simulink model "MPC_PMM_ph_gaslift"  (R2023a)
settings: Solver=ode15s  StartTime=0.0  StopTime=par.simulation_time  FixedStep=par.sample_time  RelTol=1e-3
values from neighbouring files (symbols this model uses):
  A = blkdiag(plant_discrete.A, plant_output_disturbance.A)    [main_MPC_PMM_ph_gaslift.m]
  Bu = [plant_discrete.B; 0]    [main_MPC_PMM_ph_gaslift.m]
  Cm = [plant_discrete.C, plant_output_disturbance.C]    [main_MPC_PMM_ph_gaslift.m]
  par = function_parameters_MPC_PMM_ph_gaslift    [main_MPC_PMM_ph_gaslift.m]
  u0 = operating_report.Inputs.u    [main_MPC_PMM_ph_gaslift.m]
  x0 = [operating_report.States(1).x; operating_report.States(2).x]    [main_MPC_PMM_ph_gaslift.m]
  y0 = operating_report.Outputs.y    [main_MPC_PMM_ph_gaslift.m]
undefined symbols (not defined in the file or in its folder): L, M
libraries: mpclib x1
settings Model: ExtModeTrigMode=oneshot  Creator=The MathWorks, Inc.  LastModifiedBy=aslik
settings SolverCC: ZeroCrossControl=DisableAll  ZeroCrossAlgorithm=Adaptive  AlgebraicLoopSolver=TrustRegion
settings DataIOCC: InspectSignalLogs=on  ReturnWorkspaceOutputs=off  DatasetSignalFormat=timetable
settings OptimizationCC: BooleanDataType=off  DefaultParameterBehavior=Inlined  EnhancedBackFolding=on  PassReuseOutputArgsAs=Individual arguments  ExpressionDepthLimit=2147483647  ZeroExternalMemoryAtStartup=off  ZeroInternalMemoryAtStartup=off  InitFltsAndDblsToZero=on  OptimizeBlockOrder=speed  DifferentSizesBufferReuse=on  OptimizationCustomize=off  EfficientTunableParamExpr=on
settings DebuggingCC: UnderspecifiedInitializationDetection=Classic  MergeDetectMultiDrivingBlocksExec=none  CheckExecutionContextPreStartOutputMsg=on  SignalResolutionControl=TryResolveAllWithWarning  IgnoredZcDiagnostic=none  MultiTaskDSMMsg=warning  MultiTaskCondExecSysMsg=none  IntegerOverflowMsg=none  ParameterTunabilityLossMsg=error  FcnCallInpInsideContextMsg=warning  UnconnectedInputMsg=warning  UnconnectedOutputMsg=warning  UnconnectedLineMsg=warning  StateNameClashWarn=warning  SFUnexpectedBacktrackingDiag=warning  SFNoUnconditionalDefaultTransitionDiag=warning  SFExecutionAtInitializationDiag=none  IntegerSaturationMsg=none  ArithmeticOperatorsInVariantConditions=warning
settings HardwareCC: TargetBitPerPointer=64  TargetBitPerSizeT=64  TargetBitPerPtrDiffT=64  TargetLongLongMode=on  TargetIntDivRoundTo=Zero  TargetEndianess=LittleEndian  TargetWordSize=64  TargetHWDeviceType=MATLAB Host  ProdEqTarget=off
settings ModelReferenceCC: EnableRefExpFcnMdlSchedulingChecks=on  PropagateSignalLabelsOutOfModel=off
settings SFSimCC: SimUseLocalCustomCode=off  MATLABDynamicMemAlloc=off  CustomCodeUndefinedFunction=UseInterfaceOnly
settings RTWCC: Description=Embedded Coder  SystemTargetFile=ert.tlc  TemplateMakefile=ert_default_tmf  RTWUseLocalCustomCode=off  DLArmComputeVersion=19.05
settings CodeAppCC: ForceParamTrailComments=on  IgnoreCustomStorageClasses=off  OperatorAnnotations=on  SimulinkDataObjDesc=on  SFDataObjDesc=on  InsertBlockDesc=on
settings ERTTargetCC: GenerateSampleERTMain=on  InlinedParameterPlacement=NonHierarchical  ERTCustomFileTemplate=example_file_process.tlc
settings ConfigComp: CovMetricSettings=dw  CovSaveCumulativeToWorkspaceVar=on  CovSaveSingleToWorkspaceVar=on  CovExternalEMLEnable=off  CovSFcnEnable=off

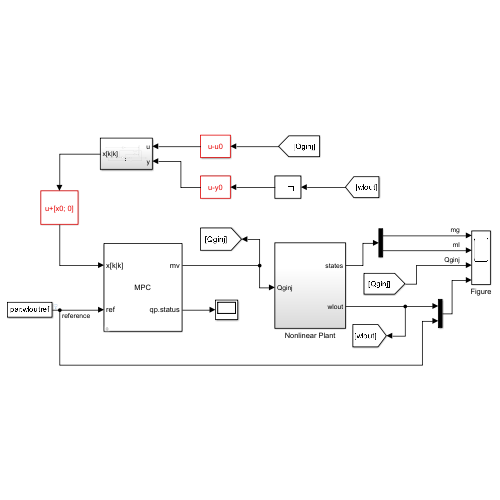
[thumbnail: Simulink's stored preview of the top-level diagram]
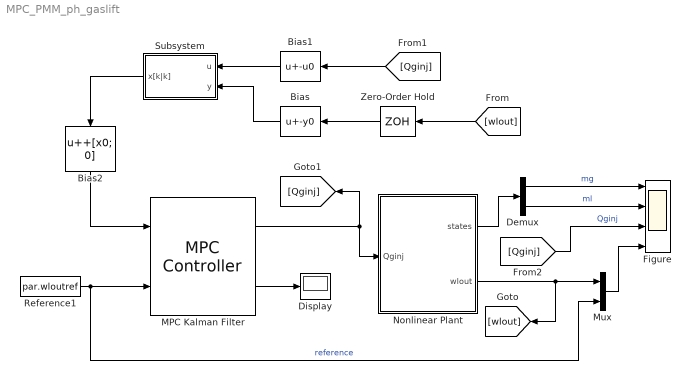
== system MPC_PMM_ph_gaslift ==
  Bias : Bias  Bias=-y0  SaturateOnIntegerOverflow=off
  Bias1 : Bias  Bias=-u0  SaturateOnIntegerOverflow=off
  Bias2 : Bias  Bias=+[x0; 0]  SaturateOnIntegerOverflow=off
  Demux : Demux  Outputs=2
  Display : Display
  Figure : Scope  NumInputPorts=4
  MPC Kalman Filter : mpclib/MPC Controller  mpcobj=mpcobj  x0=[]  is_multiple=0  enable_value=0  return_u0=off  updateMPCinCallerWorkspace=on  md_inport=off  mv_inport=off  uref_inport=off  return_cost=off  return_mvseq=off  return_qpstatus=on  return_xseq=off  return_state=off  return_ovseq=off  state_inport=on  umin_inport=off  umax_inport=off  ymin_inport=off  ymax_inport=off  cc_inport=off  ywt_inport=off  uwt_inport=off  duwt_inport=off  rhoeps_inport=off  pm_inport=off  MaximumP=10  HorizonChoice=FixedHorizon  n_ts=0.01  n_p=10  n_mv=1  n_md=0  n_ud=0  n_mo=1  n_uo=0  BlockDataType=double  SampleTimeInherited=off  switch_inport=off
  Mux : Mux  Inputs=2
  Nonlinear Plant : Subsystem
  Reference1 : Constant  Value=par.wloutref  SampleTime=0
  Subsystem : Subsystem
  Zero-Order Hold : ZeroOrderHold  SampleTime=par.sample_time
  wires:
  Bias/1 -> Subsystem/2(y)
  Nonlinear Plant/2(wlout) -> [wlout], Mux/1
  Reference1/1 -> MPC Kalman Filter/2, Mux/2  "reference"
  Bias2/1 -> MPC Kalman Filter/1
  Bias1/1 -> Subsystem/1(u)
  MPC Kalman Filter/1 -> Nonlinear Plant/1(Qginj), [Qginj]
  Zero-Order Hold/1 -> Bias/1
  Subsystem/1(x[k|k]) -> Bias2/1
  [Qginj] -> Figure/3  "Qginj"
  [Qginj] -> Bias1/1
  Nonlinear Plant/1(states) -> Demux/1
  Demux/2 -> Figure/2  "ml"
  Demux/1 -> Figure/1  "mg"
  [wlout] -> Zero-Order Hold/1
  Mux/1 -> Figure/4
  MPC Kalman Filter/2 -> Display/1

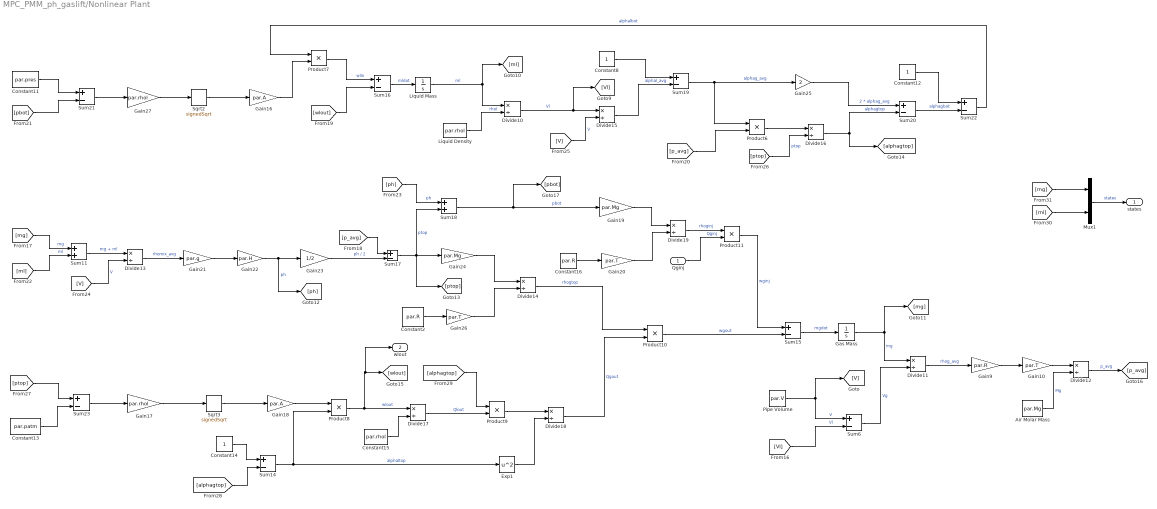
== system MPC_PMM_ph_gaslift/Nonlinear Plant ==
  Qginj : Inport
  Air Molar Mass : Constant  Value=par.Mg  OutDataTypeStr=double
  Constant11 : Constant  Value=par.pres  OutDataTypeStr=double
  Constant12 : Constant  OutDataTypeStr=double
  Constant13 : Constant  Value=par.patm  OutDataTypeStr=double
  Constant14 : Constant  OutDataTypeStr=double
  Constant15 : Constant  Value=par.rhol  OutDataTypeStr=double
  Constant16 : Constant  Value=par.R  OutDataTypeStr=double
  Constant2 : Constant  Value=par.R  OutDataTypeStr=double
  Constant8 : Constant  OutDataTypeStr=double
  Divide{10..19} (10 alike) : Product  Inputs=*/
  Exp1 : Math  Operator=square
  Gain10 : Gain  Gain=par.T
  Gain16 : Gain  Gain=par.A
  Gain17 : Gain  Gain=par.rhol
  Gain18 : Gain  Gain=par.A
  Gain19 : Gain  Gain=par.Mg
  Gain20 : Gain  Gain=par.T
  Gain21 : Gain  Gain=par.g
  Gain22 : Gain  Gain=par.H
  Gain23 : Gain  Gain=1/2
  Gain24 : Gain  Gain=par.Mg
  Gain25 : Gain  Gain=2
  Gain26 : Gain  Gain=par.T
  Gain27 : Gain  Gain=par.rhol
  Gain9 : Gain  Gain=par.R
  "Gas Mass " : Integrator  InitialCondition=x0(1)  LowerSaturationLimit=0  ContinuousStateAttributes='mg'
  Liquid Density : Constant  Value=par.rhol  OutDataTypeStr=double
  Liquid Mass : Integrator  InitialCondition=x0(2)  LowerSaturationLimit=0  ContinuousStateAttributes='ml'
  Mux1 : Mux  Inputs=2
  Pipe Volume : Constant  Value=par.V  OutDataTypeStr=double
  Product{6..11} (6 alike) : Product
  Sqrt2 : Sqrt  Operator=signedSqrt
  Sqrt3 : Sqrt  Operator=signedSqrt
  Sum11 : Sum
  Sum{6,14..17,19..23} (10 alike) : Sum  Inputs=+-
  Sum18 : Sum
  states : Outport
  wlout : Outport  Port=2
  wires:
  Liquid Mass/1 -> [ml], Divide10/1  "ml"
  Constant13/1 -> Sum23/2
  Sum6/1 -> Divide11/2  "Vg"
  Sum11/1 -> Divide13/1  "mg + ml"
  Gain18/1 -> Product8/1
  Product7/1 -> Sum16/1  "wlin"
  Product10/1 -> Sum15/2  "wgout"
  "Gas Mass "/1 -> [mg], Divide11/1  "mg"
  Gain22/1 -> [ph], Gain23/1  "ph"
  [mg] -> Sum11/1  "mg"
  [ml] -> Sum11/2  "ml"
  Sqrt2/1 -> Gain16/1
  [wlout] -> Sum16/2
  [V] -> Divide13/2  "V"
  Air Molar Mass/1 -> Divide12/2  "Mg"
  Sum18/1 -> [pbot], Gain19/1  "pbot"
  Divide19/1 -> Product11/1  "rhoginj"
  Product9/1 -> Divide18/1
  Sum20/1 -> Sum22/2  "alphagbot"
  [pbot] -> Sum21/2
  Constant2/1 -> Gain26/1
  Liquid Density/1 -> Divide10/2  "rhol"
  Sqrt3/1 -> Gain18/1
  Sum19/1 -> Product6/1, Gain25/1  "alphag_avg"
  [ptop] -> Divide16/2  "ptop"
  Constant12/1 -> Sum22/1
  Qginj/1 -> Product11/2  "Qginj"
  [alphagtop] -> Product9/1
  Sum15/1 -> "Gas Mass "/1  "mgdot"
  Gain24/1 -> Divide14/1
  Gain23/1 -> Sum17/2  "ph / 2"
  [p_avg] -> Sum17/1
  [Vl] -> Sum6/2  "Vl"
  Sum21/1 -> Gain27/1
  Divide18/1 -> Product10/2  "Qgout"
  Gain9/1 -> Gain10/1
  Divide13/1 -> Gain21/1  "rhomix_avg"
  Gain27/1 -> Sqrt2/1
  Gain26/1 -> Divide14/2
  Exp1/1 -> Divide18/2
  Product11/1 -> Sum15/1  "wginj"
  Gain25/1 -> Sum20/1  "2 * alphag_avg"
  Pipe Volume/1 -> [V], Sum6/1  "V"
  [p_avg] -> Product6/2
  Constant11/1 -> Sum21/1
  Gain10/1 -> Divide12/1
  Gain20/1 -> Divide19/2
  Sum17/1 -> Gain24/1, Sum18/2, [ptop]  "ptop"
  Sum14/1 -> Product8/2, Exp1/1  "alphaltop"
  Divide15/1 -> Sum19/2  "alphal_avg"
  Gain19/1 -> Divide19/1
  Product6/1 -> Divide16/1
  Divide12/1 -> [p_avg]  "p_avg"
  Gain16/1 -> Product7/2
  Product8/1 -> wlout/1, [wlout], Divide17/1  "wlout"
  Constant14/1 -> Sum14/1
  [ml] -> Mux1/2
  Sum23/1 -> Gain17/1
  Constant15/1 -> Divide17/2
  [mg] -> Mux1/1
  Divide11/1 -> Gain9/1  "rhog_avg"
  Mux1/1 -> states/1  "states"
  Divide14/1 -> Product10/1  "rhogtop"
  Sum16/1 -> Liquid Mass/1  "mldot"
  [V] -> Divide15/2  "V"
  [alphagtop] -> Sum14/2
  Gain17/1 -> Sqrt3/1
  Gain21/1 -> Gain22/1
  Constant8/1 -> Sum19/1
  Constant16/1 -> Gain20/1
  Divide17/1 -> Product9/2  "Qlout"
  [ph] -> Sum18/1  "ph"
  Divide16/1 -> [alphagtop], Sum20/2  "alphagtop"
  Divide10/1 -> Divide15/1, [Vl]  "Vl"
  Sum22/1 -> Product7/1  "alphalbot"
  [ptop] -> Sum23/1

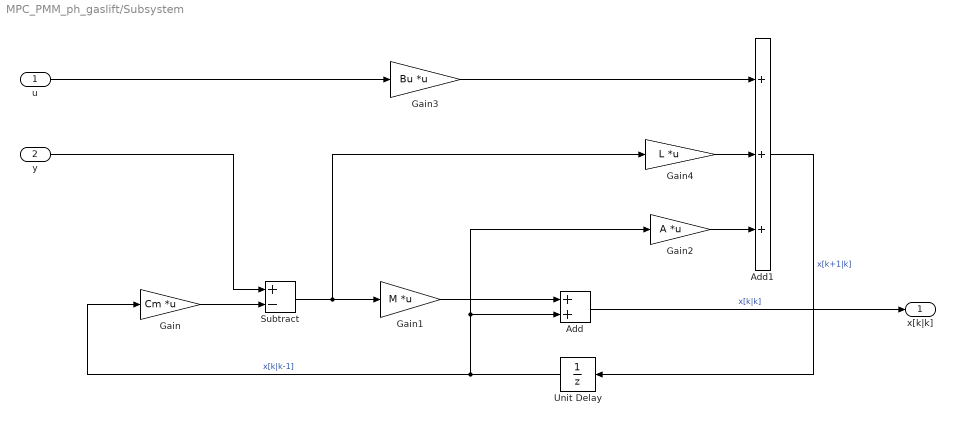
== system MPC_PMM_ph_gaslift/Subsystem ==
  u : Inport
  y : Inport  Port=2
  Add : Sum
  Add1 : Sum  Inputs=+++
  Gain : Gain  Gain=Cm  Multiplication=Matrix(K*u)
  Gain1 : Gain  Gain=M  Multiplication=Matrix(K*u)
  Gain2 : Gain  Gain=A  Multiplication=Matrix(K*u)
  Gain3 : Gain  Gain=Bu  Multiplication=Matrix(K*u)
  Gain4 : Gain  Gain=L  Multiplication=Matrix(K*u)
  Subtract : Sum  Inputs=+-
  Unit Delay : UnitDelay  InitialCondition=zeros(3,1)  SampleTime=par.sample_time  HasFrameUpgradeWarning=on
  x[k|k] : Outport  VectorParamsAs1DForOutWhenUnconnected=off
  wires:
  Unit Delay/1 -> Gain/1, Gain2/1, Add/2  "x[k|k-1]"
  Gain1/1 -> Add/1
  Add1/1 -> Unit Delay/1  "x[k+1|k]"
  Add/1 -> x[k|k]/1  "x[k|k]"
  Gain/1 -> Subtract/2
  Gain4/1 -> Add1/2
  Gain2/1 -> Add1/3
  Gain3/1 -> Add1/1
  u/1 -> Gain3/1
  y/1 -> Subtract/1
  Subtract/1 -> Gain4/1, Gain1/1
